simulink model "TestNozzleChoked"  (R2019b)
settings: Solver=ode45  StartTime=0.0  StopTime=10.0  RelTol=1e-3  EnableMultiTasking=on
libraries: Lib_TurboC_FlowStart_TMATSC x1, Lib_TurboC_Nozzle_TMATSC x1
settings Model: Creator=tlavelle  LastModifiedBy=bhisma
settings DataIOCC: LimitDataPoints=on  SaveFormat=Array  ReturnWorkspaceOutputs=off
settings OptimizationCC: ExpressionDepthLimit=2147483647  LifeSpan=inf
settings DebuggingCC: UnderspecifiedInitializationDetection=Classic  MergeDetectMultiDrivingBlocksExec=none  SolverPrmCheckMsg=warning  StateNameClashWarn=warning  SFUnexpectedBacktrackingDiag=warning  SFNoUnconditionalDefaultTransitionDiag=warning  SFExecutionAtInitializationDiag=none  ArithmeticOperatorsInVariantConditions=warning
settings HardwareCC: ProdBitPerPointer=32  ProdBitPerSizeT=32  ProdBitPerPtrDiffT=32  ProdLargestAtomicFloat=None  ProdIntDivRoundTo=Undefined  ProdEndianess=Unspecified  ProdWordSize=32  ProdHWDeviceType=32-bit Generic
settings ModelReferenceCC: PropagateSignalLabelsOutOfModel=off
settings SFSimCC: SimUseLocalCustomCode=off  CustomCodeUndefinedFunction=UseInterfaceOnly
settings RTWCC: RTWUseLocalCustomCode=off
settings CodeAppCC: StateflowObjectComments=on
settings GRTTargetCC: TargetLangStandard=C89/C90 (ANSI)  GeneratePreprocessorConditionals=Disable all
settings ConfigComp: CovMetricSettings=dw  CovHtmlReporting=on  CovSaveCumulativeToWorkspaceVar=on  CovSaveSingleToWorkspaceVar=on  CovExternalEMLEnable=off

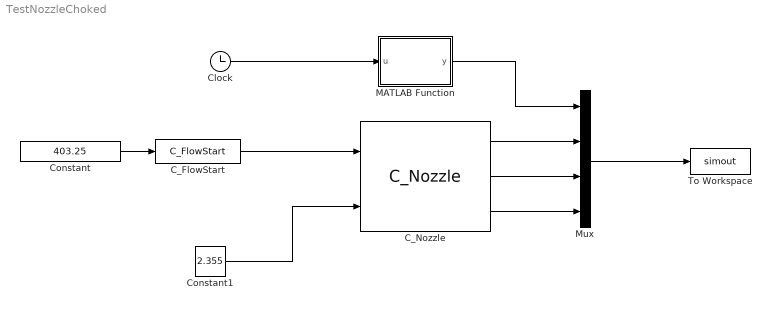
== system TestNozzleChoked ==
  C_FlowStart : Lib_TurboC_FlowStart_TMATSC/C_FlowStart  Tt_M=533.3  Pt_M=6.47  comp1_M=1  comp2_M=0  comp3_M=0  comp4_M=0  comp5_M=0  comp6_M=0
  C_Nozzle : Lib_TurboC_Nozzle_TMATSC/C_Nozzle  Ath_in_M=2706.36  Cfg_M=.9975  IDes_M=2  Wdes_M=366.66
  Clock : Clock
  Constant : Constant  Value=403.25
  Constant1 : Constant  Value=2.355
  MATLAB Function : MATLAB Function  TreatAsAtomicUnit=on
  Mux : Mux
  To Workspace : ToWorkspace  VariableName=simout  SaveFormat=Timeseries  SampleTime=-1
  wires:
  Constant/1 -> C_FlowStart/1
  C_FlowStart/1 -> C_Nozzle/1
  Constant1/1 -> C_Nozzle/2
  Clock/1 -> MATLAB Function/1(u)
  MATLAB Function/1(y) -> Mux/1
  C_Nozzle/1 -> Mux/2
  C_Nozzle/2 -> Mux/3
  C_Nozzle/3 -> Mux/4
  Mux/1 -> To Workspace/1

== matlab function TestNozzleChoked/MATLAB Function ==
  data: u input; y output
function y = fcn(u)
%#codegen
eml.extrinsic('set_param');
if u < 3
   set_param('TestNozzleChoked/C_Nozzle','IDes_M','0');
elseif u< 6 
   set_param('TestNozzleChoked/C_Nozzle','IDes_M','1'); 
else 
   set_param('TestNozzleChoked/C_Nozzle','IDes_M','2'); 
end    
y = u;
